simulink model "q_1"  (R2022a)
settings: Solver=VariableStepAuto  StartTime=0.0  StopTime=0.05  RelTol=1e-3
undefined symbols (not defined in the file or in its folder): D1, Delta, lagging, pulse
libraries: spsSeriesRLCBranchLib x33, spsGroundLib x8, spsUniversalBridgeLib x4, spsPLL3phLib x2, spsPulseGeneratorThyristor12PulseLib x2, spsThreePhaseVIMeasurementLib x2, spsThreePhaseTransformerThreeWindingsLib x2, spsThreePhaseSourceLib x2, spsCurrentMeasurementLib x1, spspowerguiLib x1
settings Model: Creator=mianyangdashu  LastModifiedBy=ds
settings DataIOCC: ReturnWorkspaceOutputs=off
settings DebuggingCC: UnconnectedInputMsg=warning  UnconnectedOutputMsg=warning  UnconnectedLineMsg=warning
settings RTWCC: DLArmComputeVersion=19.05

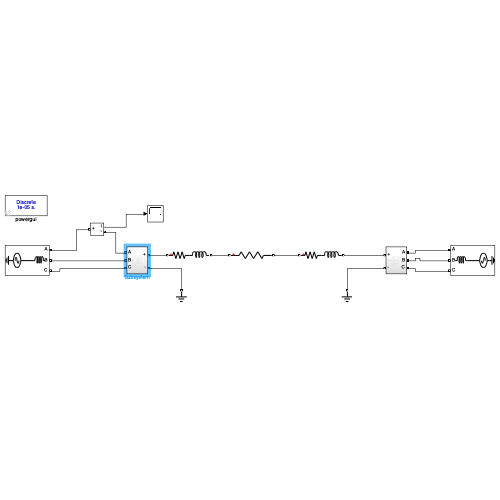
[thumbnail: Simulink's stored preview of the top-level diagram]
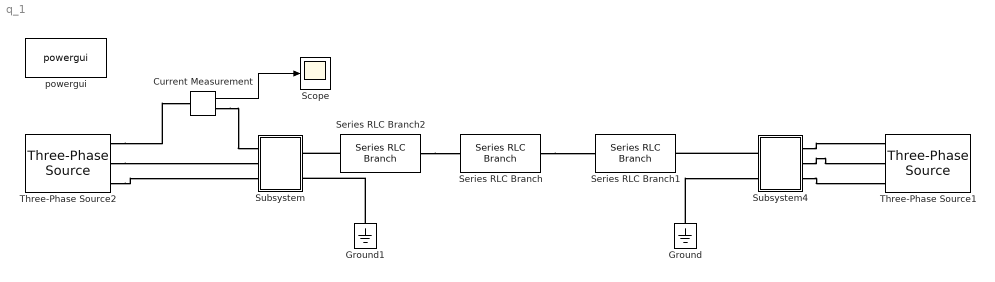
== system q_1 ==
  Current Measurement : spsCurrentMeasurementLib/Current Measurement  PhasorSimulation=off  OutputType=Complex  PSBequivalent=0
  Ground : spsGroundLib/Ground  LConnTagsString=a
  Ground1 : spsGroundLib/Ground  LConnTagsString=a
  Scope : Scope
  Series RLC Branch : spsSeriesRLCBranchLib/Series RLC Branch  LConnTagsString=__new0  RConnTagsString=__new0  BranchType=R  Resistance=250  Inductance=0.5  SetiL0=off  InitialCurrent=0  Capacitance=0  Setx0=off  InitialVoltage=0  Measurements=None
  Series RLC Branch1 : spsSeriesRLCBranchLib/Series RLC Branch  LConnTagsString=__new0  RConnTagsString=__new0  BranchType=RL  Resistance=0  Inductance=0.5  SetiL0=off  InitialCurrent=0  Capacitance=0  Setx0=off  InitialVoltage=0  Measurements=None
  Series RLC Branch2 : spsSeriesRLCBranchLib/Series RLC Branch  LConnTagsString=__new0  RConnTagsString=__new0  BranchType=RL  Resistance=0  Inductance=0.5  SetiL0=off  InitialCurrent=0  Capacitance=0  Setx0=off  InitialVoltage=0  Measurements=None
  Subsystem : Subsystem
  Subsystem4 : Subsystem
  Three-Phase Source1 : spsThreePhaseSourceLib/Three-Phase Source  InternalConnection=Yg  VoltagePhases=off  Voltage=345e3  PhaseAngle=0  Voltage_phases=[25e3 25e3 25e3]/sqrt(3)  PhaseAngles_phases=[0 -120 +120]  Frequency=50  NonIdealSource=on  SpecifyImpedance=off  Resistance=0  Inductance=16.58e-3  ShortCircuitLevel=100e6  BaseVoltage=25e3  XRratio=7  BusType=swing  Pref=10e3  Qref=0  Prefabc=[10e3, 10e3, 10e3]  Qrefabc=[0, 0, 0]  Qmin=-inf  Qmax=inf
  Three-Phase Source2 : spsThreePhaseSourceLib/Three-Phase Source  InternalConnection=Yg  VoltagePhases=off  Voltage=345e3  PhaseAngle=0  Voltage_phases=[25e3 25e3 25e3]/sqrt(3)  PhaseAngles_phases=[0 -120 +120]  Frequency=50  NonIdealSource=on  SpecifyImpedance=off  Resistance=0  Inductance=16.03e-3  ShortCircuitLevel=100e6  BaseVoltage=0  XRratio=7  BusType=swing  Pref=10e3  Qref=0  Prefabc=[10e3, 10e3, 10e3]  Qrefabc=[0, 0, 0]  Qmin=-inf  Qmax=inf
  powergui : spspowerguiLib/powergui  Priority=1  SimulationMode=Discrete  SampleTime=1e-5  frequency=60  Iterations=50  frequencyindice=50  Pbase=100e6  ErrMax=1e-4  UnitsV=kV  UnitsW=MW  buscounter=0  FunctionMessages=off  echomessages=off  EnableUseOfTLC=off  CurrentSourceSwitches=off  DisableSnubberDevices=off  DisableRonSwitches=off  DisableVfSwitches=off  DisplayEquations=off  AutomaticDiscreteSolvers=off  SolverType=Tustin/Backward Euler (TBE)  Interpol=off  ExternalGateDelay=off  methode=off  Ts=100  x0status=blocks  SPID=on  SwTol=0  HookPort=off  NonlinearTolerance=1e-4  nMaxIteration=100  ContinueOnMaxIteration=off  RestoreLinks=warning  ResistiveCurrentMeasurement=off  Frange=[0:2:500]  Ylog=off  Xlog=on  ShowGrid=off  save=off  variable=ZData  structure=0  ZoomFFT=off  StartTime=0.0  cycles=1  DisplayStyle=1  fundamental=60  FreqAxis=off  MaxFrequency=1000  frequencyindicesteady=1  RmsSteady=1  display=off
  wires:
  Current Measurement/1 -> Scope/1
  connections:
  Three-Phase Source2/RConn1 -- Current Measurement/LConn1
  Three-Phase Source2/RConn2 -- Subsystem/LConn2
  Three-Phase Source2/RConn3 -- Subsystem/LConn3
  Subsystem4/LConn1 -- Three-Phase Source1/RConn1
  Subsystem4/LConn2 -- Three-Phase Source1/RConn2
  Subsystem4/LConn3 -- Three-Phase Source1/RConn3
  Series RLC Branch2/LConn1 -- Subsystem/RConn1
  Subsystem4/RConn1 -- Series RLC Branch1/RConn1
  Ground/LConn1 -- Subsystem4/RConn2
  Current Measurement/RConn1 -- Subsystem/LConn1
  Ground1/LConn1 -- Subsystem/RConn2
  Series RLC Branch/RConn1 -- Series RLC Branch1/LConn1
  Series RLC Branch2/RConn1 -- Series RLC Branch/LConn1

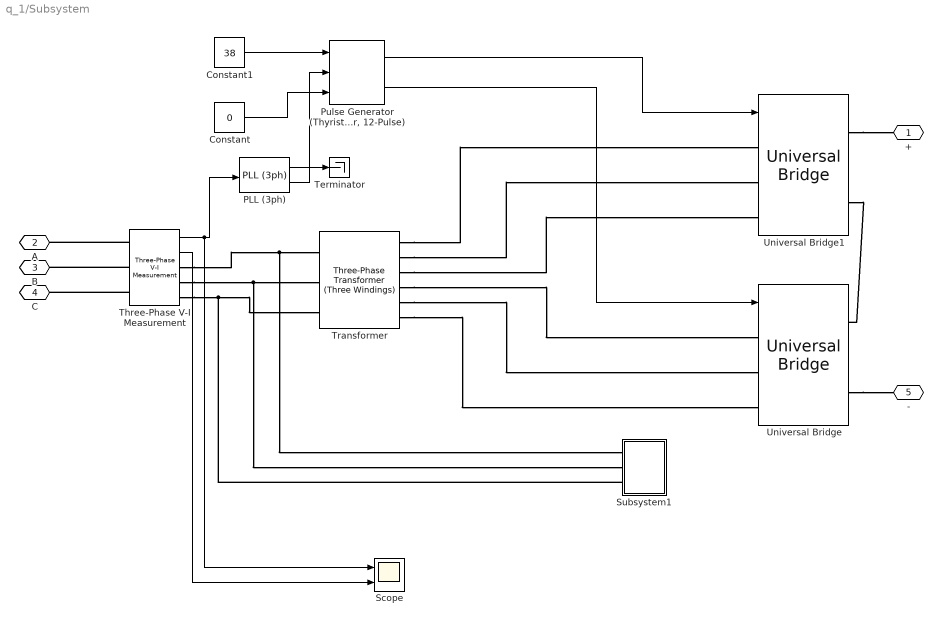
== system q_1/Subsystem ==
  Constant : Constant  Value=0
  Constant1 : Constant  Value=38
  PLL (3ph) : spsPLL3phLib/PLL (3ph)  Fmin=50  Par_Init=[0, 50]  ParK=[180, 3200, 1]  TcD=1e-4  MaxRateChangeFreq=12  FilterCutOffFreq=25  Ts=0  AGC=on
  "Pulse Generator (Thyristor, 12-Pulse)" : spsPulseGeneratorThyristor12PulseLib/Pulse Generator (Thyristor, 12-Pulse)  GenType=12-pulse  Delta=D1 (lagging)  pwidth=60  Double_Pulse=off  Ts=50e-6
      settings: SourceProductBaseCode=PS
  Scope : Scope  NumInputPorts=2
  Subsystem1 : Subsystem
  Terminator : Terminator
  Three-Phase V-I Measurement : spsThreePhaseVIMeasurementLib/Three-Phase V-I Measurement  VoltageMeasurement=phase-to-ground  SetLabelV=off  LabelV=Vabc  Vpu=off  VpuLL=off  CurrentMeasurement=yes  SetLabelI=off  LabelI=Iabc  Ipu=off  Pbase=100e6  Vbase=500e3  OutputType=Complex  PhasorSimulation=off  PSBequivalent=0
  "Transformer " : spsThreePhaseTransformerThreeWindingsLib/Three-Phase Transformer (Three Windings)  Winding1Connection=Yg  Winding2Connection=Y  Winding3Connection=Delta (D1)  CoreType=Three single-phase transformers  SetSaturation=off  Hysteresis=off  DataFile='hysteresis'  SetInitialFlux=off  Measurements=Winding currents  UNITS=pu  NominalPower=[ 1200e6 , 50 ]  Winding1=[ 345e3 , 0.002 , 0.08 ]  Winding2=[ 200e3 , 0.002 , 0.08 ]  Winding3=[ 200e3 , 0.002 , 0.08 ]  Rm=500  Lm=500  L0=0.5  Saturation=[ 0,0 ; 0.0024,1.2 ; 1.0,1.52 ]  InitialFluxes=[0.8 -0.8 0.7]  BreakLoop=off  DiscreteSolver=Trapezoidal iterative  DataType=off  TransfoNumber=1
      settings: SourceProductBaseCode=PS
  Universal Bridge : spsUniversalBridgeLib/Universal Bridge  Arms=3  SnubberResistance=1e5  SnubberCapacitance=inf  Device=Thyristors  Ron=1e-3  Lon=0  ForwardVoltages="[  0  0  ]"  ForwardVoltage=0  GTOparameters=[ 10e-6 , 20e-6 ]  IGBTparameters=[ 1e-6 , 2e-6 ]  Measurements=None  Measurements_2=None  converterType=Rectifier
  Universal Bridge1 : spsUniversalBridgeLib/Universal Bridge  Arms=3  SnubberResistance=1e5  SnubberCapacitance=inf  Device=Thyristors  Ron=1e-3  Lon=0  ForwardVoltages="[  0  0  ]"  ForwardVoltage=0  GTOparameters=[ 10e-6 , 20e-6 ]  IGBTparameters=[ 1e-6 , 2e-6 ]  Measurements=None  Measurements_2=None  converterType=Rectifier
  + : PMIOPort  Side=Right
  A : PMIOPort  Port=2  Side=Left
  B : PMIOPort  Port=3  Side=Left
  C : PMIOPort  Port=4  Side=Left
  - : PMIOPort  Port=5  Side=Right
  wires:
  Three-Phase V-I Measurement/1 -> Scope/1, PLL (3ph)/1
  "Pulse Generator (Thyristor, 12-Pulse)"/2 -> Universal Bridge/1
  PLL (3ph)/2 -> "Pulse Generator (Thyristor, 12-Pulse)"/2
  "Pulse Generator (Thyristor, 12-Pulse)"/1 -> Universal Bridge1/1
  PLL (3ph)/1 -> Terminator/1
  Three-Phase V-I Measurement/2 -> Scope/2
  Constant/1 -> "Pulse Generator (Thyristor, 12-Pulse)"/3
  Constant1/1 -> "Pulse Generator (Thyristor, 12-Pulse)"/1
  connections:
  Three-Phase V-I Measurement/LConn3 -- C/RConn1
  "Transformer "/RConn1 -- Universal Bridge1/LConn1
  "Transformer "/RConn4 -- Universal Bridge/LConn1
  Three-Phase V-I Measurement/LConn2 -- B/RConn1
  "Transformer "/RConn6 -- Universal Bridge/LConn3
  Universal Bridge/RConn2 -- -/RConn1
  Universal Bridge1/RConn1 -- +/RConn1
  Universal Bridge1/RConn2 -- Universal Bridge/RConn1
  "Transformer "/RConn2 -- Universal Bridge1/LConn2
  Three-Phase V-I Measurement/LConn1 -- A/RConn1
  "Transformer "/RConn3 -- Universal Bridge1/LConn3
  "Transformer "/RConn5 -- Universal Bridge/LConn2
  Three-Phase V-I Measurement/RConn2 -- Subsystem1/LConn2 -- "Transformer "/LConn2
  Three-Phase V-I Measurement/RConn1 -- Subsystem1/LConn1 -- "Transformer "/LConn1
  Three-Phase V-I Measurement/RConn3 -- Subsystem1/LConn3 -- "Transformer "/LConn3

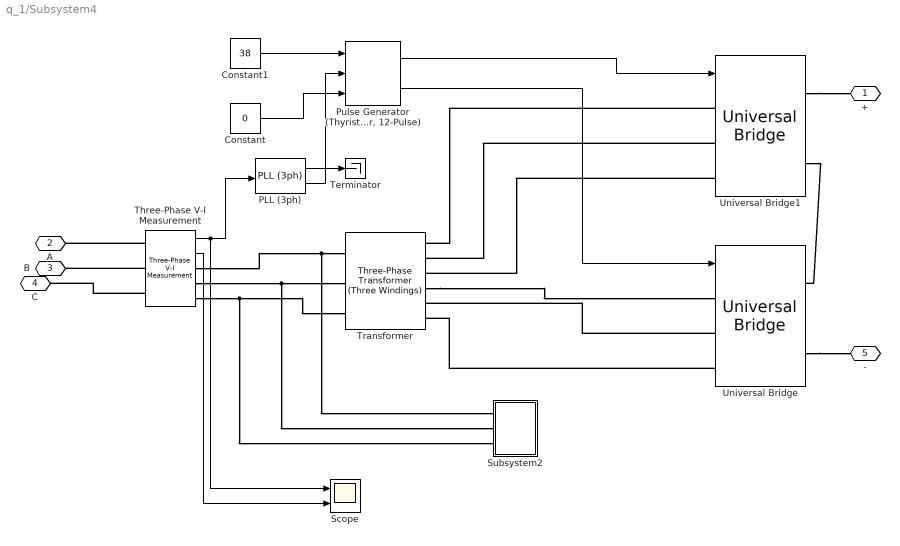
== system q_1/Subsystem4 ==
  Constant : Constant  Value=0
  Constant1 : Constant  Value=38
  PLL (3ph) : spsPLL3phLib/PLL (3ph)  Fmin=50  Par_Init=[0, 50]  ParK=[180, 3200, 1]  TcD=1e-4  MaxRateChangeFreq=12  FilterCutOffFreq=25  Ts=0  AGC=on
  "Pulse Generator (Thyristor, 12-Pulse)" : spsPulseGeneratorThyristor12PulseLib/Pulse Generator (Thyristor, 12-Pulse)  GenType=12-pulse  Delta=D1 (lagging)  pwidth=60  Double_Pulse=off  Ts=0
      settings: SourceProductBaseCode=PS
  Scope : Scope  NumInputPorts=2
  Subsystem2 : Subsystem
  Terminator : Terminator
  Three-Phase V-I Measurement : spsThreePhaseVIMeasurementLib/Three-Phase V-I Measurement  VoltageMeasurement=phase-to-ground  SetLabelV=off  LabelV=Vabc  Vpu=off  VpuLL=off  CurrentMeasurement=yes  SetLabelI=off  LabelI=Iabc  Ipu=off  Pbase=100e6  Vbase=500e3  OutputType=Complex  PhasorSimulation=off  PSBequivalent=0
  "Transformer " : spsThreePhaseTransformerThreeWindingsLib/Three-Phase Transformer (Three Windings)  Winding1Connection=Yg  Winding2Connection=Y  Winding3Connection=Delta (D1)  CoreType=Three single-phase transformers  SetSaturation=off  Hysteresis=off  DataFile='hysteresis'  SetInitialFlux=off  Measurements=Winding currents  UNITS=pu  NominalPower=[ 1200e6 , 50 ]  Winding1=[ 345e3 , 0.002 , 0.08 ]  Winding2=[ 200e3 , 0.002 , 0.08 ]  Winding3=[ 200e3 , 0.002 , 0.08 ]  Rm=500  Lm=500  L0=0.5  Saturation=[ 0,0 ; 0.0024,1.2 ; 1.0,1.52 ]  InitialFluxes=[0.8 -0.8 0.7]  BreakLoop=off  DiscreteSolver=Trapezoidal iterative  DataType=off  TransfoNumber=1
      settings: SourceProductBaseCode=PS
  Universal Bridge : spsUniversalBridgeLib/Universal Bridge  Arms=3  SnubberResistance=1e5  SnubberCapacitance=inf  Device=Thyristors  Ron=1e-3  Lon=0  ForwardVoltages="[  0  0  ]"  ForwardVoltage=0  GTOparameters=[ 10e-6 , 20e-6 ]  IGBTparameters=[ 1e-6 , 2e-6 ]  Measurements=None  Measurements_2=None  converterType=Rectifier
  Universal Bridge1 : spsUniversalBridgeLib/Universal Bridge  Arms=3  SnubberResistance=1e5  SnubberCapacitance=inf  Device=Thyristors  Ron=1e-3  Lon=0  ForwardVoltages="[  0  0  ]"  ForwardVoltage=0  GTOparameters=[ 10e-6 , 20e-6 ]  IGBTparameters=[ 1e-6 , 2e-6 ]  Measurements=None  Measurements_2=None  converterType=Rectifier
  + : PMIOPort  Side=Right
  A : PMIOPort  Port=2  Side=Left
  B : PMIOPort  Port=3  Side=Left
  C : PMIOPort  Port=4  Side=Left
  - : PMIOPort  Port=5  Side=Right
  wires:
  Three-Phase V-I Measurement/1 -> Scope/1, PLL (3ph)/1
  "Pulse Generator (Thyristor, 12-Pulse)"/2 -> Universal Bridge/1
  PLL (3ph)/2 -> "Pulse Generator (Thyristor, 12-Pulse)"/2
  Constant/1 -> "Pulse Generator (Thyristor, 12-Pulse)"/3
  "Pulse Generator (Thyristor, 12-Pulse)"/1 -> Universal Bridge1/1
  PLL (3ph)/1 -> Terminator/1
  Three-Phase V-I Measurement/2 -> Scope/2
  Constant1/1 -> "Pulse Generator (Thyristor, 12-Pulse)"/1
  connections:
  Three-Phase V-I Measurement/LConn3 -- C/RConn1
  Universal Bridge1/LConn1 -- "Transformer "/RConn1
  "Transformer "/RConn4 -- Universal Bridge/LConn1
  Three-Phase V-I Measurement/LConn2 -- B/RConn1
  Universal Bridge/LConn3 -- "Transformer "/RConn6
  Universal Bridge/RConn2 -- -/RConn1
  Universal Bridge1/RConn1 -- +/RConn1
  Universal Bridge1/RConn2 -- Universal Bridge/RConn1
  Three-Phase V-I Measurement/LConn1 -- A/RConn1
  Universal Bridge1/LConn2 -- "Transformer "/RConn2
  Universal Bridge1/LConn3 -- "Transformer "/RConn3
  Universal Bridge/LConn2 -- "Transformer "/RConn5
  Three-Phase V-I Measurement/RConn2 -- Subsystem2/LConn2 -- "Transformer "/LConn2
  Three-Phase V-I Measurement/RConn1 -- Subsystem2/LConn1 -- "Transformer "/LConn1
  Three-Phase V-I Measurement/RConn3 -- Subsystem2/LConn3 -- "Transformer "/LConn3

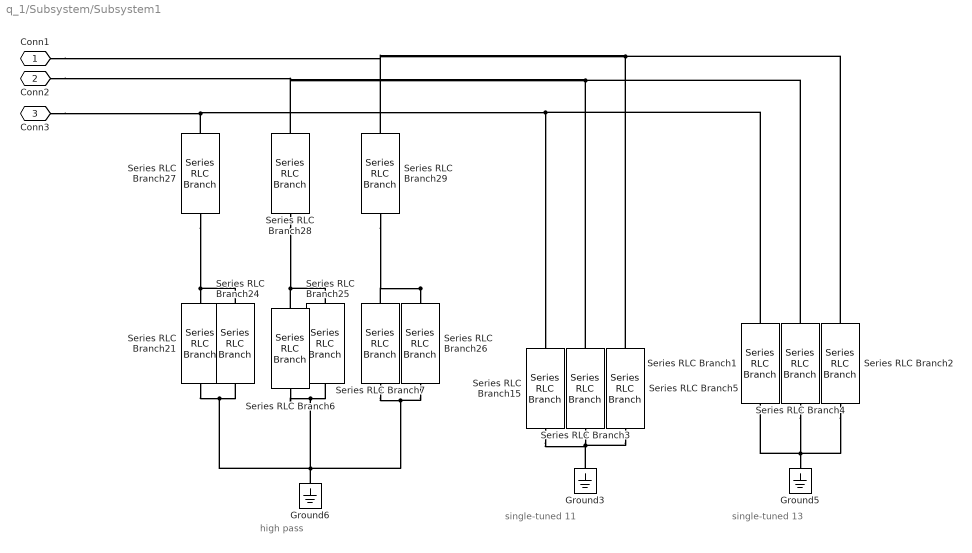
== system q_1/Subsystem/Subsystem1 ==
  note: single-tuned 11
  note: high pass
  note: single-tuned 13
  Ground3 : spsGroundLib/Ground  LConnTagsString=a
  Ground5 : spsGroundLib/Ground  LConnTagsString=a
  Ground6 : spsGroundLib/Ground  LConnTagsString=a
  Series RLC Branch1 : spsSeriesRLCBranchLib/Series RLC Branch  LConnTagsString=__new0  RConnTagsString=__new0  BranchType=RLC  Resistance=0.9156  Inductance=22.4e-3  SetiL0=off  InitialCurrent=0  Capacitance=2.6743e-6  Setx0=off  InitialVoltage=0  Measurements=None
  Series RLC Branch15 : spsSeriesRLCBranchLib/Series RLC Branch  LConnTagsString=__new0  RConnTagsString=__new0  BranchType=RLC  Resistance=1.0820  Inductance=31.3e-3  SetiL0=off  InitialCurrent=0  Capacitance=2.6743e-6  Setx0=off  InitialVoltage=0  Measurements=None
  Series RLC Branch2 : spsSeriesRLCBranchLib/Series RLC Branch  LConnTagsString=__new0  RConnTagsString=__new0  BranchType=RLC  Resistance=0.9156  Inductance=22.4e-3  SetiL0=off  InitialCurrent=0  Capacitance=2.6743e-6  Setx0=off  InitialVoltage=0  Measurements=None
  Series RLC Branch21 : spsSeriesRLCBranchLib/Series RLC Branch  LConnTagsString=__new0  RConnTagsString=__new0  BranchType=L  Resistance=1  Inductance=0.1579e-3  SetiL0=off  InitialCurrent=0  Capacitance=0.1114e-6  Setx0=off  InitialVoltage=0  Measurements=None
  Series RLC Branch24 : spsSeriesRLCBranchLib/Series RLC Branch  LConnTagsString=__new0  RConnTagsString=__new0  BranchType=R  Resistance=1190.25  Inductance=1e-3  SetiL0=off  InitialCurrent=0  Capacitance=1e-6  Setx0=off  InitialVoltage=0  Measurements=None
  Series RLC Branch25 : spsSeriesRLCBranchLib/Series RLC Branch  LConnTagsString=__new0  RConnTagsString=__new0  BranchType=R  Resistance=1190.25  Inductance=1e-3  SetiL0=off  InitialCurrent=0  Capacitance=1e-6  Setx0=off  InitialVoltage=0  Measurements=None
  Series RLC Branch26 : spsSeriesRLCBranchLib/Series RLC Branch  LConnTagsString=__new0  RConnTagsString=__new0  BranchType=R  Resistance=1190.25  Inductance=1e-3  SetiL0=off  InitialCurrent=0  Capacitance=1e-6  Setx0=off  InitialVoltage=0  Measurements=None
  Series RLC Branch27 : spsSeriesRLCBranchLib/Series RLC Branch  LConnTagsString=__new0  RConnTagsString=__new0  BranchType=C  Resistance=1  Inductance=1e-3  SetiL0=off  InitialCurrent=0  Capacitance=0.1114e-6  Setx0=off  InitialVoltage=0  Measurements=None
  Series RLC Branch28 : spsSeriesRLCBranchLib/Series RLC Branch  LConnTagsString=__new0  RConnTagsString=__new0  BranchType=C  Resistance=1  Inductance=1e-3  SetiL0=off  InitialCurrent=0  Capacitance=0.1114e-6  Setx0=off  InitialVoltage=0  Measurements=None
  Series RLC Branch29 : spsSeriesRLCBranchLib/Series RLC Branch  LConnTagsString=__new0  RConnTagsString=__new0  BranchType=C  Resistance=1  Inductance=1e-3  SetiL0=off  InitialCurrent=0  Capacitance=0.1114e-6  Setx0=off  InitialVoltage=0  Measurements=None
  Series RLC Branch3 : spsSeriesRLCBranchLib/Series RLC Branch  LConnTagsString=__new0  RConnTagsString=__new0  BranchType=RLC  Resistance=1.0820  Inductance=31.3e-3  SetiL0=off  InitialCurrent=0  Capacitance=2.6743e-6  Setx0=off  InitialVoltage=0  Measurements=None
  Series RLC Branch4 : spsSeriesRLCBranchLib/Series RLC Branch  LConnTagsString=__new0  RConnTagsString=__new0  BranchType=RLC  Resistance=0.9156  Inductance=22.4e-3  SetiL0=off  InitialCurrent=0  Capacitance=2.6743e-6  Setx0=off  InitialVoltage=0  Measurements=None
  Series RLC Branch5 : spsSeriesRLCBranchLib/Series RLC Branch  LConnTagsString=__new0  RConnTagsString=__new0  BranchType=RLC  Resistance=1.0820  Inductance=31.3e-3  SetiL0=off  InitialCurrent=0  Capacitance=2.6743e-6  Setx0=off  InitialVoltage=0  Measurements=None
  Series RLC Branch6 : spsSeriesRLCBranchLib/Series RLC Branch  LConnTagsString=__new0  RConnTagsString=__new0  BranchType=L  Resistance=1  Inductance=0.1579e-3  SetiL0=off  InitialCurrent=0  Capacitance=0.1114e-6  Setx0=off  InitialVoltage=0  Measurements=None
  Series RLC Branch7 : spsSeriesRLCBranchLib/Series RLC Branch  LConnTagsString=__new0  RConnTagsString=__new0  BranchType=L  Resistance=1  Inductance=0.1579e-3  SetiL0=off  InitialCurrent=0  Capacitance=0.1114e-6  Setx0=off  InitialVoltage=0  Measurements=None
  Conn1 : PMIOPort  Side=Left
  Conn2 : PMIOPort  Port=2  Side=Left
  Conn3 : PMIOPort  Port=3  Side=Left
  connections:
  Series RLC Branch4/LConn1 -- Series RLC Branch1/LConn1 -- Ground5/LConn1 -- Series RLC Branch2/LConn1
  Series RLC Branch26/LConn1 -- Series RLC Branch29/RConn1 -- Series RLC Branch7/LConn1
  Series RLC Branch26/RConn1 -- Ground6/LConn1 -- Series RLC Branch6/RConn1 -- Series RLC Branch25/RConn1 -- Series RLC Branch21/RConn1 -- Series RLC Branch24/RConn1 -- Series RLC Branch7/RConn1
  Series RLC Branch4/RConn1 -- Series RLC Branch28/LConn1 -- Conn2/RConn1 -- Series RLC Branch3/RConn1
  Series RLC Branch25/LConn1 -- Series RLC Branch28/RConn1 -- Series RLC Branch6/LConn1
  Series RLC Branch24/LConn1 -- Series RLC Branch21/LConn1 -- Series RLC Branch27/RConn1
  Series RLC Branch27/LConn1 -- Conn3/RConn1 -- Series RLC Branch15/RConn1 -- Series RLC Branch1/RConn1
  Series RLC Branch3/LConn1 -- Series RLC Branch15/LConn1 -- Ground3/LConn1 -- Series RLC Branch5/LConn1
  Series RLC Branch2/RConn1 -- Series RLC Branch29/LConn1 -- Conn1/RConn1 -- Series RLC Branch5/RConn1

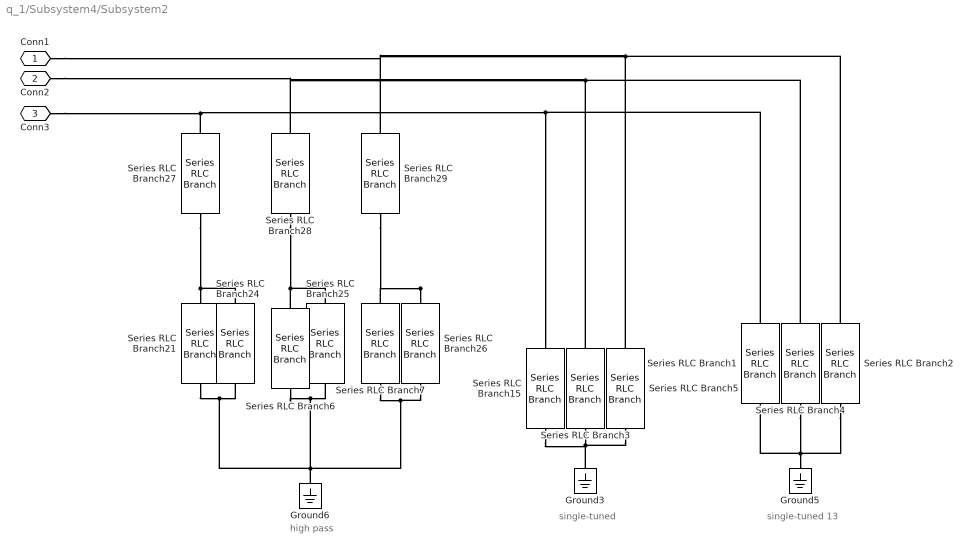
== system q_1/Subsystem4/Subsystem2 ==
  note: single-tuned
  note: high pass
  note: single-tuned 13
  Ground3 : spsGroundLib/Ground  LConnTagsString=a
  Ground5 : spsGroundLib/Ground  LConnTagsString=a
  Ground6 : spsGroundLib/Ground  LConnTagsString=a
  Series RLC Branch1 : spsSeriesRLCBranchLib/Series RLC Branch  LConnTagsString=__new0  RConnTagsString=__new0  BranchType=RLC  Resistance=0.9156  Inductance=22.4e-3  SetiL0=off  InitialCurrent=0  Capacitance=2.6743e-6  Setx0=off  InitialVoltage=0  Measurements=None
  Series RLC Branch15 : spsSeriesRLCBranchLib/Series RLC Branch  LConnTagsString=__new0  RConnTagsString=__new0  BranchType=RLC  Resistance=1.0820  Inductance=31.3e-3  SetiL0=off  InitialCurrent=0  Capacitance=2.6743e-6  Setx0=off  InitialVoltage=0  Measurements=None
  Series RLC Branch2 : spsSeriesRLCBranchLib/Series RLC Branch  LConnTagsString=__new0  RConnTagsString=__new0  BranchType=RLC  Resistance=0.9156  Inductance=22.4e-3  SetiL0=off  InitialCurrent=0  Capacitance=2.6743e-6  Setx0=off  InitialVoltage=0  Measurements=None
  Series RLC Branch21 : spsSeriesRLCBranchLib/Series RLC Branch  LConnTagsString=__new0  RConnTagsString=__new0  BranchType=L  Resistance=1  Inductance=0.1579e-3  SetiL0=off  InitialCurrent=0  Capacitance=0.1114e-6  Setx0=off  InitialVoltage=0  Measurements=None
  Series RLC Branch24 : spsSeriesRLCBranchLib/Series RLC Branch  LConnTagsString=__new0  RConnTagsString=__new0  BranchType=R  Resistance=1190.25  Inductance=1e-3  SetiL0=off  InitialCurrent=0  Capacitance=1e-6  Setx0=off  InitialVoltage=0  Measurements=None
  Series RLC Branch25 : spsSeriesRLCBranchLib/Series RLC Branch  LConnTagsString=__new0  RConnTagsString=__new0  BranchType=R  Resistance=1190.25  Inductance=1e-3  SetiL0=off  InitialCurrent=0  Capacitance=1e-6  Setx0=off  InitialVoltage=0  Measurements=None
  Series RLC Branch26 : spsSeriesRLCBranchLib/Series RLC Branch  LConnTagsString=__new0  RConnTagsString=__new0  BranchType=R  Resistance=1190.25  Inductance=1e-3  SetiL0=off  InitialCurrent=0  Capacitance=1e-6  Setx0=off  InitialVoltage=0  Measurements=None
  Series RLC Branch27 : spsSeriesRLCBranchLib/Series RLC Branch  LConnTagsString=__new0  RConnTagsString=__new0  BranchType=C  Resistance=1  Inductance=1e-3  SetiL0=off  InitialCurrent=0  Capacitance=0.1114e-6  Setx0=off  InitialVoltage=0  Measurements=None
  Series RLC Branch28 : spsSeriesRLCBranchLib/Series RLC Branch  LConnTagsString=__new0  RConnTagsString=__new0  BranchType=C  Resistance=1  Inductance=1e-3  SetiL0=off  InitialCurrent=0  Capacitance=0.1114e-6  Setx0=off  InitialVoltage=0  Measurements=None
  Series RLC Branch29 : spsSeriesRLCBranchLib/Series RLC Branch  LConnTagsString=__new0  RConnTagsString=__new0  BranchType=C  Resistance=1  Inductance=1e-3  SetiL0=off  InitialCurrent=0  Capacitance=0.1114e-6  Setx0=off  InitialVoltage=0  Measurements=None
  Series RLC Branch3 : spsSeriesRLCBranchLib/Series RLC Branch  LConnTagsString=__new0  RConnTagsString=__new0  BranchType=RLC  Resistance=1.0820  Inductance=31.3e-3  SetiL0=off  InitialCurrent=0  Capacitance=2.6743e-6  Setx0=off  InitialVoltage=0  Measurements=None
  Series RLC Branch4 : spsSeriesRLCBranchLib/Series RLC Branch  LConnTagsString=__new0  RConnTagsString=__new0  BranchType=RLC  Resistance=0.9156  Inductance=22.4e-3  SetiL0=off  InitialCurrent=0  Capacitance=2.6743e-6  Setx0=off  InitialVoltage=0  Measurements=None
  Series RLC Branch5 : spsSeriesRLCBranchLib/Series RLC Branch  LConnTagsString=__new0  RConnTagsString=__new0  BranchType=RLC  Resistance=1.0820  Inductance=31.3e-3  SetiL0=off  InitialCurrent=0  Capacitance=2.6743e-6  Setx0=off  InitialVoltage=0  Measurements=None
  Series RLC Branch6 : spsSeriesRLCBranchLib/Series RLC Branch  LConnTagsString=__new0  RConnTagsString=__new0  BranchType=L  Resistance=1  Inductance=0.1579e-3  SetiL0=off  InitialCurrent=0  Capacitance=0.1114e-6  Setx0=off  InitialVoltage=0  Measurements=None
  Series RLC Branch7 : spsSeriesRLCBranchLib/Series RLC Branch  LConnTagsString=__new0  RConnTagsString=__new0  BranchType=L  Resistance=1  Inductance=0.1579e-3  SetiL0=off  InitialCurrent=0  Capacitance=0.1114e-6  Setx0=off  InitialVoltage=0  Measurements=None
  Conn1 : PMIOPort  Side=Left
  Conn2 : PMIOPort  Port=2  Side=Left
  Conn3 : PMIOPort  Port=3  Side=Left
  connections:
  Series RLC Branch4/LConn1 -- Series RLC Branch1/LConn1 -- Ground5/LConn1 -- Series RLC Branch2/LConn1
  Series RLC Branch26/LConn1 -- Series RLC Branch29/RConn1 -- Series RLC Branch7/LConn1
  Series RLC Branch26/RConn1 -- Ground6/LConn1 -- Series RLC Branch6/RConn1 -- Series RLC Branch25/RConn1 -- Series RLC Branch21/RConn1 -- Series RLC Branch24/RConn1 -- Series RLC Branch7/RConn1
  Series RLC Branch4/RConn1 -- Series RLC Branch28/LConn1 -- Conn2/RConn1 -- Series RLC Branch3/RConn1
  Series RLC Branch25/LConn1 -- Series RLC Branch28/RConn1 -- Series RLC Branch6/LConn1
  Series RLC Branch24/LConn1 -- Series RLC Branch21/LConn1 -- Series RLC Branch27/RConn1
  Series RLC Branch27/LConn1 -- Conn3/RConn1 -- Series RLC Branch15/RConn1 -- Series RLC Branch1/RConn1
  Series RLC Branch3/LConn1 -- Series RLC Branch15/LConn1 -- Ground3/LConn1 -- Series RLC Branch5/LConn1
  Series RLC Branch2/RConn1 -- Series RLC Branch29/LConn1 -- Conn1/RConn1 -- Series RLC Branch5/RConn1
